simulink model "ngc"  (R2020b)
settings: Solver=VariableStepAuto  StartTime=0.0  StopTime=90  RelTol=1e-3
values from neighbouring files (symbols this model uses):
  A = [-1.064 1.000;290.26 0.00]    [model.m]
  B = [-0.25; -331.40]    [model.m]
  C = [-123.34 0.00; 0.00 1.00]    [model.m]
  D = [-13.51; 0]    [model.m]
  dT1 = 0.75    [model.m]
  dT2 = 0.25    [model.m]
  ELEV_INIT = 10000    [model.m]
  ELEV_TARGET = 21    [model.m]
  LAT_INIT = 36.161748    [model.m]
  LAT_OBS = 35.423623    [model.m]
  LAT_TARGET = 35.375527    [model.m]
  LON_INIT = 139.2982418    [model.m]
  LON_OBS = 139.48858    [model.m]
  LON_TARGET = 139.525105    [model.m]
  Vel = 1021.08    [model.m]
undefined symbols (not defined in the file or in its folder): Earth, K, L, WGS84
libraries: simulink x3, aerolibtransform2 x1, pid_lib x1, aerolibanimutils x1
settings Model: Creator=shohei  LastModifiedBy=shohei

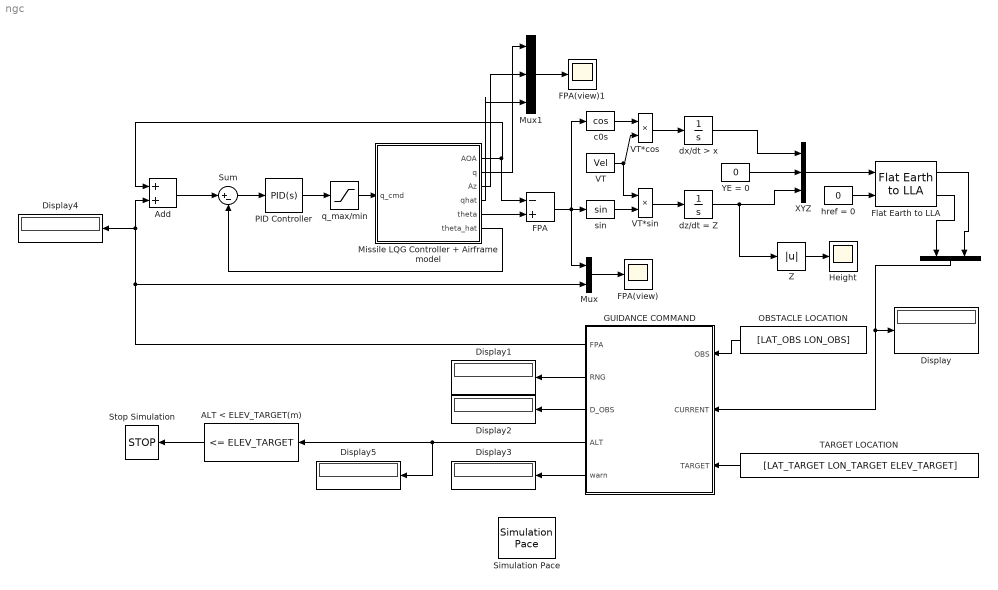
== system ngc ==
  " " : Mux  Inputs=2
  ALT < ELEV_TARGET(m) : simulink/Logic and Bit Operations/Compare To Constant  relop=<=  const=ELEV_TARGET  OutDataTypeStr=boolean
  Add : Sum
  Display{,1..5} (6 alike) : Display
  FPA : Sum  Inputs=-+
  FPA(view) : Scope
  FPA(view)1 : Scope
  Flat Earth to LLA : aerolibtransform2/Flat Earth to LLA  units=Metric (MKS)  ptype=Earth (WGS84)  F=1/298.257223563  R=6378137  refPosPort=off  LL0=[LAT_INIT LON_INIT]  psi=yaw_init
  GUIDANCE COMMAND : MATLAB Function  TreatAsAtomicUnit=on
  Height : Scope
  Missile LQG Controller + Airframe model : Subsystem
  Mux : Mux  Inputs=2
  Mux1 : Mux  Inputs=3
  OBSTACLE LOCATION : Constant  Value=[LAT_OBS LON_OBS]
  PID Controller : pid_lib/PID Controller  Controller=PID  Form=Parallel  TimeDomain=Continuous-time  UseExternalTs=off  SampleTime=-1  IntegratorMethod=Forward Euler  FilterMethod=Forward Euler  ControllerParametersSource=internal  P=-1  I=0  D=0  UseFilter=on  N=100  TunerSelectOption=Transfer Function Based (PID Tuner App)  InitialConditionSource=internal  InitialConditionForIntegrator=0  InitialConditionForFilter=0  DifferentiatorICPrevScaledInput=0  ExternalReset=none  TrackingMode=off  Kt=1  LimitOutput=off  SatLimitsSource=internal  UpperSaturationLimit=inf  LowerSaturationLimit=-inf  LinearizeAsGain=on  AntiWindupMode=none  Kb=1  POutMin=[]  POutMax=[]  IOutMin=[]  IOutMax=[]  DOutMin=[]  DOutMax=[]  NOutMin=[]  NOutMax=[]  SumOutMin=[]  SumOutMax=[]  SaturationOutMin=[]  SaturationOutMax=[]  PParamMin=[]  PParamMax=[]  IParamMin=[]  IParamMax=[]  DParamMin=[]  DParamMax=[]  NParamMin=[]  NParamMax=[]  KbParamMin=[]  KbParamMax=[]  KtParamMin=[]  KtParamMax=[]  KbOutMin=[]  KbOutMax=[]  KtOutMin=[]  KtOutMax=[]  IntegratorOutMin=[]  IntegratorOutMax=[]  FilterOutMin=[]  FilterOutMax=[]  SumI1OutMin=[]  SumI1OutMax=[]  SumI2OutMin=[]  SumI2OutMax=[]  SumI3OutMin=[]  SumI3OutMax=[]  SumI4OutMin=[]  SumI4OutMax=[]  SumDOutMin=[]  SumDOutMax=[]  DifferentiatorOutMin=[]  DifferentiatorOutMax=[]  FilterDiffOutCoefMin=[]  FilterDiffOutCoefMax=[]  ReciprocalOutMin=[]  ReciprocalOutMax=[]  SumDenOutMin=[]  SumDenOutMax=[]  SumNumOutMin=[]  SumNumOutMax=[]  DivideOutMin=[]  DivideOutMax=[]  UdiffTsProdOutMin=[]  UdiffTsProdOutMax=[]  NTsProdOutMin=[]  NTsProdOutMax=[]  UintegralTsProdOutMin=[]  UintegralTsProdOutMax=[]  UngainTsProdOutMin=[]  UngainTsProdOutMax=[]  IntegratorContinuousStateAttributes=''  IntegratorStateMustResolveToSignalObject=off  IntegratorRTWStateStorageClass=Auto  FilterContinuousStateAttributes=''  FilterStateMustResolveToSignalObject=off  FilterRTWStateStorageClass=Auto  ParallelPVariant=InternalParameters  IdealPVariant=Disabled  IVariant=InternalParameters  DVariant=InternalParameters  IntegratorVariant=Continuous  SatVariant=Disabled  AWVariant=Passthrough  PCopyVariant=Disabled  TRVariant=Disabled  FdbkBlocksVariant=Forward  IdealPFdbkVariant=Disabled  SatFdbkVariant=Disabled  DerivativeFilterVariant=ContFilter  NVariant=InternalParameters  NCopyVariant=Disabled  FilterICVariant=InternalICsFilter  IntegratorICVariant=InternalICs  ExternalResetVariant=Disabled  TRSumVariant=Passthrough  SumFdbkVariant=Disabled  SumVariant=Sum_PID  TsampFilterVariant=InternalTs  TsampNgainVariant=Passthrough  TsampIntegralVariant=Passthrough  ExternalSaturationOutDataTypeStr=Inherit: Same as second input
  Simulation Pace : aerolibanimutils/Simulation Pace  SimulationPace=2  SleepMode=MATLAB Thread  OutputPaceError=off  SampleTime=1/30
  Stop Simulation : Stop
  Sum : Sum  Inputs=|+-
  TARGET LOCATION : Constant  Value=[LAT_TARGET LON_TARGET ELEV_TARGET]
  VT : Constant  Value=Vel
  VT*cos : Product
  VT*sin : Product
  XYZ : Mux  Inputs=3
  YE = 0 : Constant  Value=0
  Z : Abs
  c0s : Trigonometry  Operator=cos
  dx/dt > x : Integrator
  dz/dt = Z : Integrator  InitialCondition=-ELEV_INIT
  href = 0 : Constant  Value=0
  q_max/min : Saturate
  sin : Trigonometry
  wires:
  PID Controller/1 -> q_max/min/1
  q_max/min/1 -> Missile LQG Controller + Airframe model/1(q_cmd)
  Missile LQG Controller + Airframe model/6(theta_hat) -> Sum/2
  Sum/1 -> PID Controller/1
  Add/1 -> Sum/1
  Missile LQG Controller + Airframe model/1(AOA) -> FPA/1, Add/1
  Missile LQG Controller + Airframe model/5(theta) -> FPA/2
  FPA/1 -> c0s/1, sin/1, Mux/1
  Mux/1 -> FPA(view)/1
  c0s/1 -> VT*cos/1
  VT/1 -> VT*sin/1, VT*cos/2
  sin/1 -> VT*sin/2
  VT*cos/1 -> dx/dt > x/1
  VT*sin/1 -> dz/dt = Z/1
  YE = 0/1 -> XYZ/2
  dx/dt > x/1 -> XYZ/1
  dz/dt = Z/1 -> Z/1, XYZ/3
  Z/1 -> Height/1
  XYZ/1 -> Flat Earth to LLA/1
  href = 0/1 -> Flat Earth to LLA/2
  Flat Earth to LLA/2 -> " "/1
  Flat Earth to LLA/1 -> " "/2
  OBSTACLE LOCATION/1 -> GUIDANCE COMMAND/1(OBS)
  TARGET LOCATION/1 -> GUIDANCE COMMAND/3(TARGET)
  " "/1 -> Display/1, GUIDANCE COMMAND/2(CURRENT)
  GUIDANCE COMMAND/2(RNG) -> Display1/1
  GUIDANCE COMMAND/3(D_OBS) -> Display2/1
  GUIDANCE COMMAND/5(warn) -> Display3/1
  GUIDANCE COMMAND/1(FPA) -> Mux/2, Display4/1, Add/2
  GUIDANCE COMMAND/4(ALT) -> Display5/1, ALT < ELEV_TARGET(m)/1
  ALT < ELEV_TARGET(m)/1 -> Stop Simulation/1
  Missile LQG Controller + Airframe model/4(qhat) -> Mux1/3
  Missile LQG Controller + Airframe model/3(Az) -> Mux1/2
  Missile LQG Controller + Airframe model/2(q) -> Mux1/1
  Mux1/1 -> FPA(view)1/1

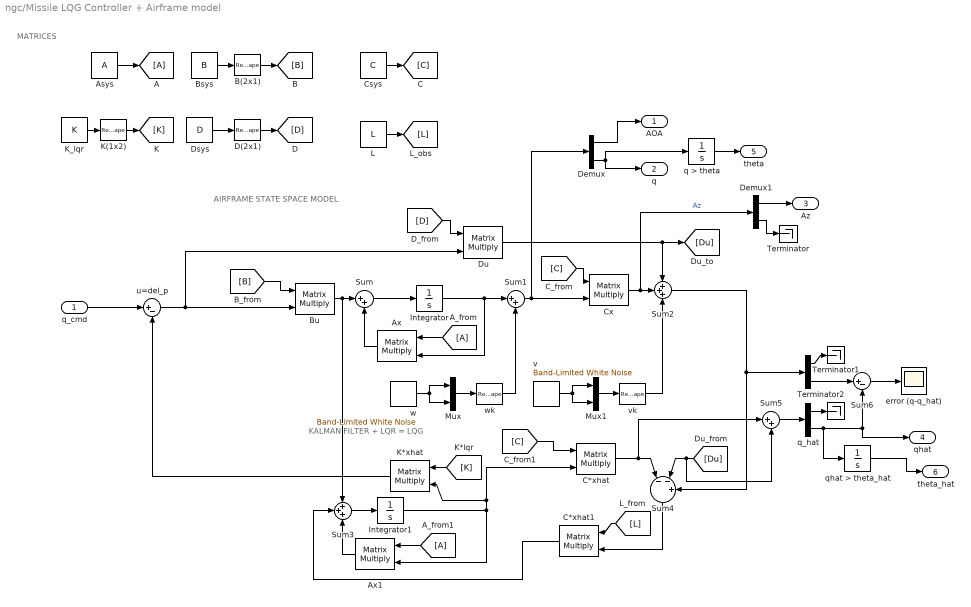
== system ngc/Missile LQG Controller + Airframe model ==
  note: KALMAN FILTER + LQR = LQG
  note: AIRFRAME STATE SPACE MODEL
  note: MATRICES
  q_cmd : Inport
  " " : Demux  Outputs=2
  Asys : Constant  Value=A
  Ax : Product  Multiplication=Matrix(*)
  Ax1 : Product  Multiplication=Matrix(*)
  B(2x1) : Reshape  OutputDimensionality=Customize  OutputDimensions=[2,1]
  "Bsys " : Constant  Value=B
  Bu : Product  Multiplication=Matrix(*)
  C*xhat : Product  Multiplication=Matrix(*)
  C*xhat1 : Product  Multiplication=Matrix(*)
  Csys : Constant  Value=C
  Cx : Product  Multiplication=Matrix(*)
  D(2x1) : Reshape  OutputDimensionality=Customize  OutputDimensions=[2,1]
  Demux : Demux  Outputs=2
  Demux1 : Demux  Outputs=2
  Dsys : Constant  Value=D
  Du : Product  Multiplication=Matrix(*)
  Integrator : Integrator
  Integrator1 : Integrator
  K(1x2) : Reshape  OutputDimensionality=Customize  OutputDimensions=[1,2]
  K*xhat : Product  Multiplication=Matrix(*)
  K_lqr : Constant  Value=K
  L : Constant  Value=L
  Mux : Mux  Inputs=2
  Mux1 : Mux  Inputs=2
  Sum : Sum  Inputs=|++
  Sum1 : Sum  Inputs=|++
  Sum2 : Sum  Inputs=+++
  Sum3 : Sum  Inputs=+++
  Sum4 : Sum  Inputs=|--+
  Sum5 : Sum  Inputs=|++
  Sum6 : Sum  Inputs=|+-
  Terminator : Terminator
  Terminator1 : Terminator
  Terminator2 : Terminator
  error (q-q_hat) : Scope
  q > theta : Integrator
  q_hat : Demux  Outputs=2
  qhat > theta_hat : Integrator
  u=del_p : Sum  Inputs=|+-
  v : simulink/Sources/Band-Limited White Noise  Cov=[0.00001]  Ts=dT2  seed=[23341]
  vk : Reshape  OutputDimensionality=Customize  OutputDimensions=[2,1]
  w : simulink/Sources/Band-Limited White Noise  Cov=[0.00000001]  Ts=dT1  seed=[23341]
  wk : Reshape  OutputDimensionality=Customize  OutputDimensions=[2,1]
  AOA : Outport
  q : Outport  Port=2
  Az : Outport  Port=3
  qhat : Outport  Port=4
  theta : Outport  Port=5
  theta_hat : Outport  Port=6
  wires:
  K_lqr/1 -> K(1x2)/1
  [K] -> K*xhat/1
  Demux1/1 -> Az/1
  q_cmd/1 -> u=del_p/1
  Demux1/2 -> Terminator/1
  q > theta/1 -> theta/1
  K(1x2)/1 -> [K]
  Demux/1 -> AOA/1
  Sum5/1 -> q_hat/1
  w/1 -> Mux/2, Mux/1
  " "/1 -> Terminator1/1
  D(2x1)/1 -> [D]
  Demux/2 -> q/1, q > theta/1
  [C] -> C*xhat/1
  [L] -> C*xhat1/1
  K*xhat/1 -> u=del_p/2
  Dsys/1 -> D(2x1)/1
  Sum4/1 -> C*xhat1/2
  Csys/1 -> [C]
  C*xhat1/1 -> Sum3/2
  Sum1/1 -> Cx/2, Demux/1
  Sum2/1 -> " "/1, Sum4/3
  [B] -> Bu/1
  Sum3/1 -> Integrator1/1
  q_hat/1 -> Terminator2/1
  u=del_p/1 -> Bu/2, Du/2
  [A] -> Ax/1
  Ax1/1 -> Sum3/3
  wk/1 -> Sum1/2
  L/1 -> [L]
  [A] -> Ax1/1
  Integrator1/1 -> C*xhat/2, K*xhat/2, Ax1/2
  vk/1 -> Sum2/3
  [C] -> Cx/1
  C*xhat/1 -> Sum5/1, Sum4/1
  [D] -> Du/1
  " "/2 -> Sum6/1
  Cx/1 -> Demux1/1, Sum2/2  "Az"
  "Bsys "/1 -> B(2x1)/1
  Bu/1 -> Sum3/1, Sum/1
  B(2x1)/1 -> [B]
  Sum/1 -> Integrator/1
  Du/1 -> [Du], Sum2/1
  [Du] -> Sum5/2, Sum4/2
  Mux/1 -> wk/1
  Mux1/1 -> vk/1
  Ax/1 -> Sum/2
  q_hat/2 -> qhat > theta_hat/1, qhat/1, Sum6/2
  Sum6/1 -> error (q-q_hat)/1
  qhat > theta_hat/1 -> theta_hat/1
  v/1 -> Mux1/2, Mux1/1
  Asys/1 -> [A]
  Integrator/1 -> Sum1/1, Ax/2

== matlab function ngc/GUIDANCE COMMAND ==
  data: OBS input; FPA output; CURRENT input; TARGET input; RNG output; D_OBS output; ALT output; warn output
function [FPA,RNG,D_OBS,ALT,warn] = fcn(OBS, CURRENT, TARGET)

R = 6371e3;
d2r = pi/180;

LAT_OBS = OBS(1);
LON_OBS = OBS(2);

thres = 2000;

LAT_TARGET = TARGET(1);
LON_TARGET = TARGET(2);
ELEV_TARGET = TARGET(3);

ELEV_CUR = CURRENT(1);
LAT_CUR = CURRENT(2);
LON_CUR = CURRENT(3);

l1 = LAT_CUR*d2r;
u1 = LON_CUR*d2r;
l2 = LAT_TARGET*d2r;
u2 = LON_TARGET*d2r;
dh = abs(ELEV_TARGET-ELEV_CUR);

dl = l2-l1;
du = u2-u1;

a = sin(dl/2)^2 + cos(l1)*cos(l2)*sin(du/2)^2;
c = 2*atan2(sqrt(a),sqrt(1-a));
d = R*c;
 
l3 = LAT_OBS*d2r;
u3 = LON_OBS*d2r;

dl = l3-l1;
du = u3-u1;

a = sin(dl/2)^2 + cos(l1)*cos(l2)*sin(du/2)^2;
c = 2*atan2(sqrt(a),sqrt(1-a));
d_obs = R*c;

range = sqrt(d^2+dh^2);

if abs(d_obs) >= thres
   w = 0;
   FPA_CMD = atan(dh/d);
else
    w = 1;
    FPA_CMD = 0;
end

FPA = FPA_CMD;
RNG = range;
D_OBS = d_obs;
warn = w;
ALT = ELEV_CUR;
